simulink model "Signals"  (Simulink 8.0)
settings: Solver=ode45  StartTime=0.0  StopTime=10.0  RelTol=1e-3
settings Model: Creator=Faradars  LastModifiedBy=Faradars

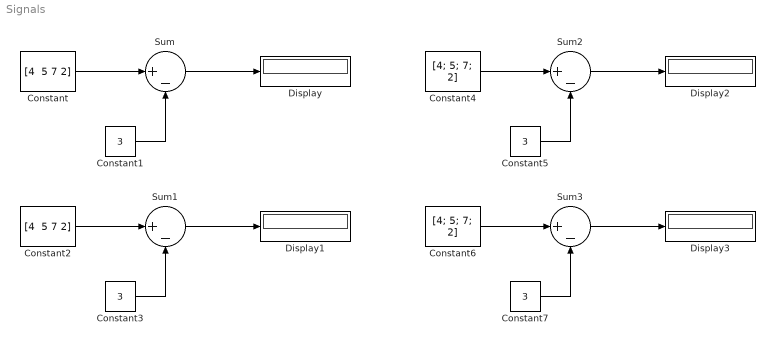
== system Signals ==
  Constant : Constant  Value="[4  5 7 2]"
  Constant{1,3,5,7} (4 alike) : Constant  Value=3
  Constant2 : Constant  Value="[4  5 7 2]"  VectorParams1D=off
  Constant4 : Constant  Value=[4; 5; 7; 2]
  Constant6 : Constant  Value=[4; 5; 7; 2]  VectorParams1D=off
  Display{,1..3} (4 alike) : Display
  Sum{,1..3} (4 alike) : Sum  Inputs=|+-
  wires:
  Constant/1 -> Sum/1
  Constant1/1 -> Sum/2
  Sum/1 -> Display/1
  Constant2/1 -> Sum1/1
  Constant3/1 -> Sum1/2
  Sum1/1 -> Display1/1
  Constant4/1 -> Sum2/1
  Constant5/1 -> Sum2/2
  Sum2/1 -> Display2/1
  Constant6/1 -> Sum3/1
  Constant7/1 -> Sum3/2
  Sum3/1 -> Display3/1
